simulink model "DALv5"  (R2021b)
settings: Solver=FixedStepAuto  StartTime=0.0  StopTime=100  RelTol=1e-3
undefined symbols (not defined in the file): Beam_Mod, magnitude, N_B, Theta_target, V_wmax
libraries: slpidlib x1
settings Model: ExtModeTrigDuration=2  Creator=Andrea  LastModifiedBy=Andrea
settings OptimizationCC: EnhancedBackFolding=on  PassReuseOutputArgsAs=Individual arguments  ZeroExternalMemoryAtStartup=off  ZeroInternalMemoryAtStartup=off  MaxStackSize=64  OptimizeBlockOrder=speed  DifferentSizesBufferReuse=on  OptimizationCustomize=off  EfficientTunableParamExpr=on
settings DebuggingCC: ParameterTunabilityLossMsg=error
settings HardwareCC: ProdBitPerInt=16  ProdBitPerPointer=16  ProdBitPerSizeT=16  ProdBitPerPtrDiffT=16  ProdLargestAtomicFloat=None  ProdWordSize=8  ProdHWDeviceType=Atmel->AVR
settings SFSimCC: MATLABDynamicMemAlloc=off
settings RTWCC: Description=Embedded Coder  SystemTargetFile=ert.tlc  HardwareBoard=Arduino Uno  TemplateMakefile=ert_default_tmf  Toolchain=Arduino AVR
settings CodeAppCC: ForceParamTrailComments=on  IgnoreCustomStorageClasses=off  OperatorAnnotations=on  SimulinkDataObjDesc=on  SFDataObjDesc=on  InsertBlockDesc=on
settings ERTTargetCC: SupportContinuousTime=on  SupportVariableSizeSignals=on  ExtModeTransport=3  ExtModeStaticAlloc=on  ExtModeStaticAllocSize=250  ExtModeMexFile=ext_xcp  ExtModeIntrfLevel=Level2 - Open

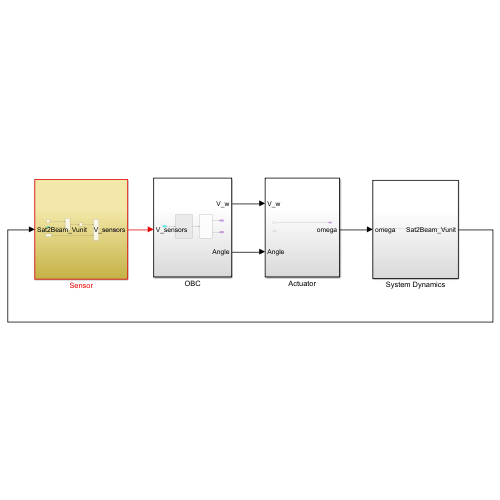
[thumbnail: Simulink's stored preview of the top-level diagram]
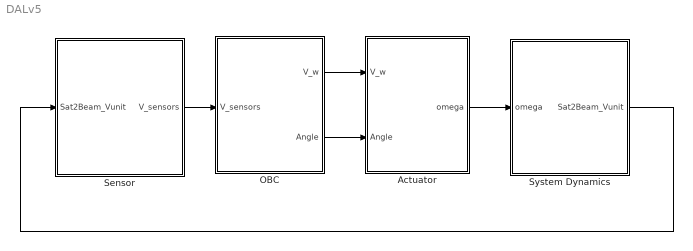
== system DALv5 ==
  Actuator : Subsystem
  OBC : Subsystem
  Sensor : Subsystem
  System Dynamics : Subsystem
  wires:
  System Dynamics/1(Sat2Beam_Vunit) -> Sensor/1(Sat2Beam_Vunit)
  Sensor/1(V_sensors) -> OBC/1(V_sensors)
  OBC/1(V_w) -> Actuator/1(V_w)
  Actuator/1(omega) -> System Dynamics/1(omega)
  OBC/2(Angle) -> Actuator/2(Angle)

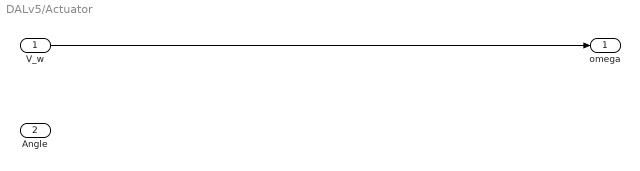
== system DALv5/Actuator ==
  V_w : Inport
  Angle : Inport  Port=2
  omega : Outport
  wires:
  V_w/1 -> omega/1

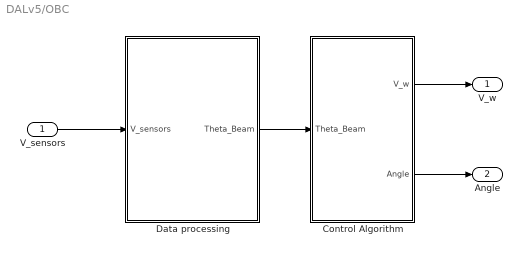
== system DALv5/OBC ==
  V_sensors : Inport
  Control Algorithm : Subsystem
  Data processing : Subsystem
  V_w : Outport
  Angle : Outport  Port=2
  wires:
  V_sensors/1 -> Data processing/1(V_sensors)
  Data processing/1(Theta_Beam) -> Control Algorithm/1(Theta_Beam)
  Control Algorithm/1(V_w) -> V_w/1
  Control Algorithm/2(Angle) -> Angle/1

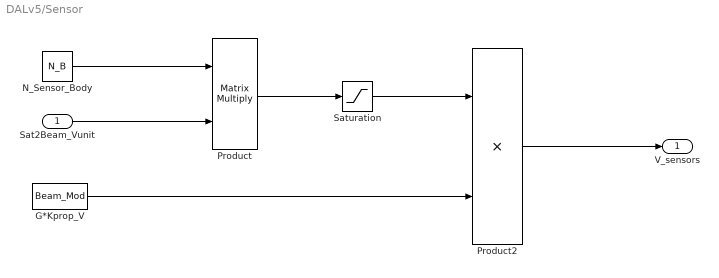
== system DALv5/Sensor ==
  Sat2Beam_Vunit : Inport
  G*Kprop_V : Constant  Value=Beam_Mod
  N_Sensor_Body : Constant  Value=N_B
  Product : Product  Multiplication=Matrix(*)
  Product2 : Product
  Saturation : Saturate  UpperLimit=1  LowerLimit=0
  V_sensors : Outport
  wires:
  Product/1 -> Saturation/1
  N_Sensor_Body/1 -> Product/1
  Saturation/1 -> Product2/1
  Product2/1 -> V_sensors/1
  Sat2Beam_Vunit/1 -> Product/2
  G*Kprop_V/1 -> Product2/2

== system DALv5/System Dynamics ==
  omega : Inport
  Sat2Beam_Vunit : Outport
  wires:
  omega/1 -> Sat2Beam_Vunit/1

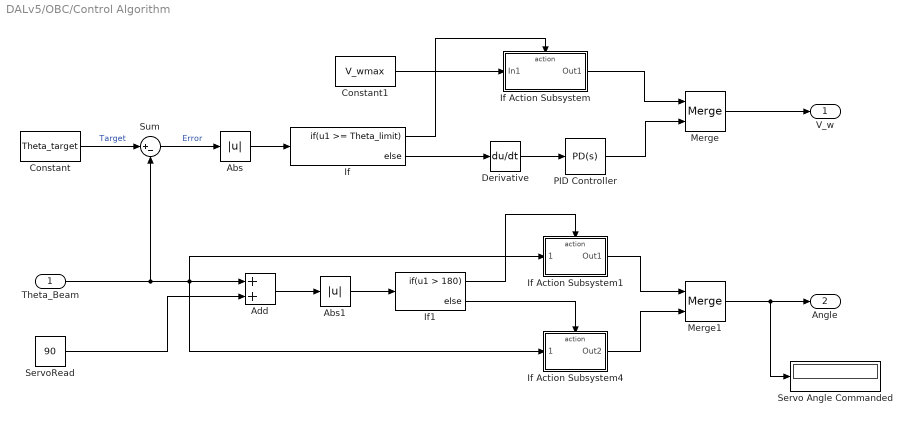
== system DALv5/OBC/Control Algorithm ==
  Theta_Beam : Inport
  Abs : Abs
  Abs1 : Abs
  Add : Sum
  Constant : Constant  Value=Theta_target
  Constant1 : Constant  Value=V_wmax
  Derivative : Derivative
  If : If  IfExpression=u1 >= Theta_limit
  If Action Subsystem : Subsystem  TreatAsAtomicUnit=on
  If Action Subsystem1 : Subsystem  TreatAsAtomicUnit=on
  If Action Subsystem4 : Subsystem  TreatAsAtomicUnit=on
  If1 : If  IfExpression=u1 > 180
  Merge : Merge
  Merge1 : Merge
  PID Controller : slpidlib/PID Controller  Controller=PD  Form=Parallel  TimeDomain=Continuous-time  UseExternalTs=off  SampleTime=-1  IntegratorMethod=Forward Euler  FilterMethod=Forward Euler  ControllerParametersSource=internal  P=1  I=1  D=0  UseFilter=on  N=100  TunerSelectOption=Transfer Function Based (PID Tuner App)  InitialConditionSource=internal  InitialConditionForIntegrator=0  InitialConditionForFilter=0  DifferentiatorICPrevScaledInput=0  ExternalReset=none  TrackingMode=off  Kt=1  LimitOutput=off  SatLimitsSource=internal  UpperSaturationLimit=inf  LowerSaturationLimit=-inf  LinearizeAsGain=on  AntiWindupMode=none  Kb=1  POutMin=[]  POutMax=[]  IOutMin=[]  IOutMax=[]  DOutMin=[]  DOutMax=[]  NOutMin=[]  NOutMax=[]  SumOutMin=[]  SumOutMax=[]  SaturationOutMin=[]  SaturationOutMax=[]  PParamMin=[]  PParamMax=[]  IParamMin=[]  IParamMax=[]  DParamMin=[]  DParamMax=[]  NParamMin=[]  NParamMax=[]  KbParamMin=[]  KbParamMax=[]  KtParamMin=[]  KtParamMax=[]  KbOutMin=[]  KbOutMax=[]  KtOutMin=[]  KtOutMax=[]  IntegratorOutMin=[]  IntegratorOutMax=[]  FilterOutMin=[]  FilterOutMax=[]  SumI1OutMin=[]  SumI1OutMax=[]  SumI2OutMin=[]  SumI2OutMax=[]  SumI3OutMin=[]  SumI3OutMax=[]  SumI4OutMin=[]  SumI4OutMax=[]  SumDOutMin=[]  SumDOutMax=[]  DifferentiatorOutMin=[]  DifferentiatorOutMax=[]  FilterDiffOutCoefMin=[]  FilterDiffOutCoefMax=[]  ReciprocalOutMin=[]  ReciprocalOutMax=[]  SumDenOutMin=[]  SumDenOutMax=[]  SumNumOutMin=[]  SumNumOutMax=[]  DivideOutMin=[]  DivideOutMax=[]  UdiffTsProdOutMin=[]  UdiffTsProdOutMax=[]  NTsProdOutMin=[]  NTsProdOutMax=[]  UintegralTsProdOutMin=[]  UintegralTsProdOutMax=[]  UngainTsProdOutMin=[]  UngainTsProdOutMax=[]  IntegratorContinuousStateAttributes=''  IntegratorStateMustResolveToSignalObject=off  IntegratorRTWStateStorageClass=Auto  FilterContinuousStateAttributes=''  FilterStateMustResolveToSignalObject=off  FilterRTWStateStorageClass=Auto  ParallelPVariant=InternalParameters  IdealPVariant=Disabled  IVariant=Disabled  DVariant=InternalParameters  IntegratorVariant=Disabled  SatVariant=Disabled  AWVariant=Disabled  PCopyVariant=Disabled  TRVariant=Disabled  FdbkBlocksVariant=Forward  IdealPFdbkVariant=Disabled  SatFdbkVariant=Disabled  DerivativeFilterVariant=ContFilter  NVariant=InternalParameters  NCopyVariant=Disabled  FilterICVariant=InternalICsFilter  IntegratorICVariant=Disabled  ExternalResetVariant=Disabled  TRSumVariant=Passthrough  SumFdbkVariant=Disabled  SumVariant=Sum_PD  TsampFilterVariant=InternalTs  TsampNgainVariant=Passthrough  TsampIntegralVariant=Disabled_SignalSpec  ExternalSaturationOutDataTypeStr=Inherit: Same as second input
  Servo Angle Commanded : Display
  ServoRead : Constant  Value=90
  Sum : Sum  Inputs=|+-
  V_w : Outport
  Angle : Outport  Port=2
  wires:
  PID Controller/1 -> Merge/2
  Constant/1 -> Sum/1  "Target"
  Sum/1 -> Abs/1  "Error"
  Constant1/1 -> If Action Subsystem/1(In1)
  If Action Subsystem/1(Out1) -> Merge/1
  If/2 -> Derivative/1
  If/1 -> If Action Subsystem/Action
  Merge/1 -> V_w/1
  Derivative/1 -> PID Controller/1
  Abs/1 -> If/1
  If1/1 -> If Action Subsystem1/Action
  Add/1 -> Abs1/1
  Merge1/1 -> Servo Angle Commanded/1, Angle/1
  Abs1/1 -> If1/1
  Theta_Beam/1 -> If Action Subsystem4/1(Light_Angle), Add/1, If Action Subsystem1/1(Light_Angle), Sum/2
  ServoRead/1 -> Add/2
  If Action Subsystem1/1(Out1) -> Merge1/1
  If1/2 -> If Action Subsystem4/Action
  If Action Subsystem4/1(Out2) -> Merge1/2

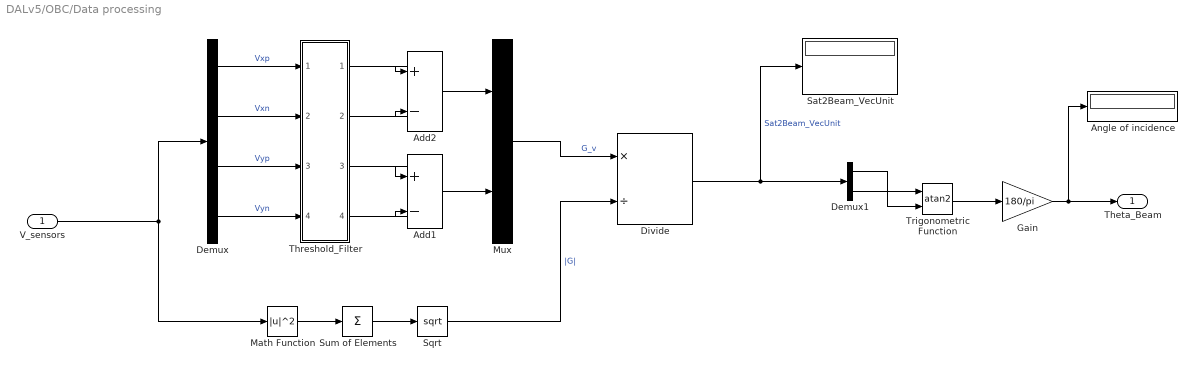
== system DALv5/OBC/Data processing ==
  V_sensors : Inport
  Add1 : Sum  Inputs=+|-
  Add2 : Sum  Inputs=+|-
  Angle of incidence : Display
  Demux : Demux
  Demux1 : Demux  Outputs=2
  Divide : Product  Inputs=*/
  Gain : Gain  Gain=180/pi
  Math Function : Math  Operator=magnitude^2  OutputSignalType=real  SaturateOnIntegerOverflow=on
  Mux : Mux  Inputs=2
  Sat2Beam_VecUnit : Display
  Sqrt : Sqrt  SaturateOnIntegerOverflow=on
  Sum of Elements : Sum  Inputs=+
  Threshold_Filter : Subsystem
  Trigonometric Function : Trigonometry  Operator=atan2
  Theta_Beam : Outport
  wires:
  Threshold_Filter/3(Out3) -> Add1/1
  Threshold_Filter/1(Out1) -> Add2/1
  Threshold_Filter/2(Out2) -> Add2/2
  Demux/4 -> Threshold_Filter/4(Vyn)  "Vyn"
  Demux/2 -> Threshold_Filter/2(Vxn)  "Vxn"
  Demux/1 -> Threshold_Filter/1(Vxp)  "Vxp"
  Demux/3 -> Threshold_Filter/3(Vyp)  "Vyp"
  Threshold_Filter/4(Out4) -> Add1/2
  Math Function/1 -> Sum of Elements/1
  Trigonometric Function/1 -> Gain/1
  Demux1/2 -> Trigonometric Function/1
  Divide/1 -> Demux1/1, Sat2Beam_VecUnit/1  "Sat2Beam_VecUnit"
  Add2/1 -> Mux/1
  Add1/1 -> Mux/2
  Demux1/1 -> Trigonometric Function/2
  Mux/1 -> Divide/1  "G_v"
  V_sensors/1 -> Math Function/1, Demux/1
  Sum of Elements/1 -> Sqrt/1
  Gain/1 -> Angle of incidence/1, Theta_Beam/1
  Sqrt/1 -> Divide/2  "|G|"

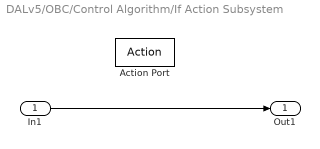
== system DALv5/OBC/Control Algorithm/If Action Subsystem ==
  In1 : Inport
  Action Port : ActionPort  ActionPortLabel=if(u1 <= Theta_limit)
  Out1 : Outport
  wires:
  In1/1 -> Out1/1

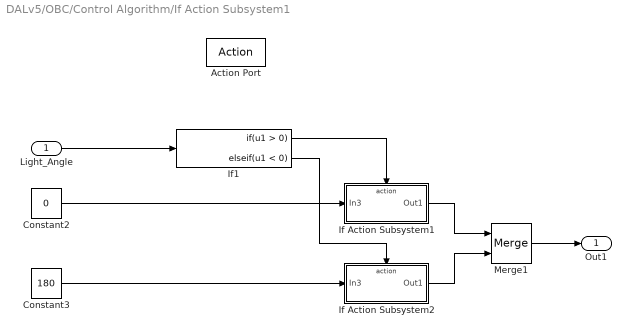
== system DALv5/OBC/Control Algorithm/If Action Subsystem1 ==
  Light_Angle : Inport
  Action Port : ActionPort  ActionPortLabel=if(u1 > 180)
  Constant2 : Constant  Value=0
  Constant3 : Constant  Value=180
  If Action Subsystem1 : Subsystem  TreatAsAtomicUnit=on
  If Action Subsystem2 : Subsystem  TreatAsAtomicUnit=on
  If1 : If  ElseIfExpressions=u1 < 0  ShowElse=off
  Merge1 : Merge
  Out1 : Outport
  wires:
  Light_Angle/1 -> If1/1
  Constant2/1 -> If Action Subsystem1/1(In3)
  Constant3/1 -> If Action Subsystem2/1(In3)
  If1/1 -> If Action Subsystem1/Action
  If1/2 -> If Action Subsystem2/Action
  Merge1/1 -> Out1/1
  If Action Subsystem1/1(Out1) -> Merge1/1
  If Action Subsystem2/1(Out1) -> Merge1/2

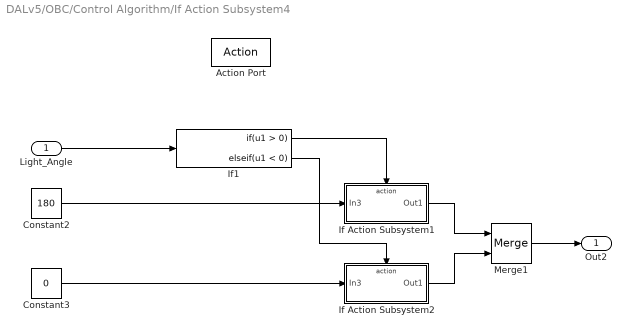
== system DALv5/OBC/Control Algorithm/If Action Subsystem4 ==
  Light_Angle : Inport
  Action Port : ActionPort  ActionPortLabel=else
  Constant2 : Constant  Value=180
  Constant3 : Constant  Value=0
  If Action Subsystem1 : Subsystem  TreatAsAtomicUnit=on
  If Action Subsystem2 : Subsystem  TreatAsAtomicUnit=on
  If1 : If  ElseIfExpressions=u1 < 0  ShowElse=off
  Merge1 : Merge
  Out2 : Outport
  wires:
  If Action Subsystem2/1(Out1) -> Merge1/2
  If1/2 -> If Action Subsystem2/Action
  Merge1/1 -> Out2/1
  Constant2/1 -> If Action Subsystem1/1(In3)
  If Action Subsystem1/1(Out1) -> Merge1/1
  Constant3/1 -> If Action Subsystem2/1(In3)
  If1/1 -> If Action Subsystem1/Action
  Light_Angle/1 -> If1/1

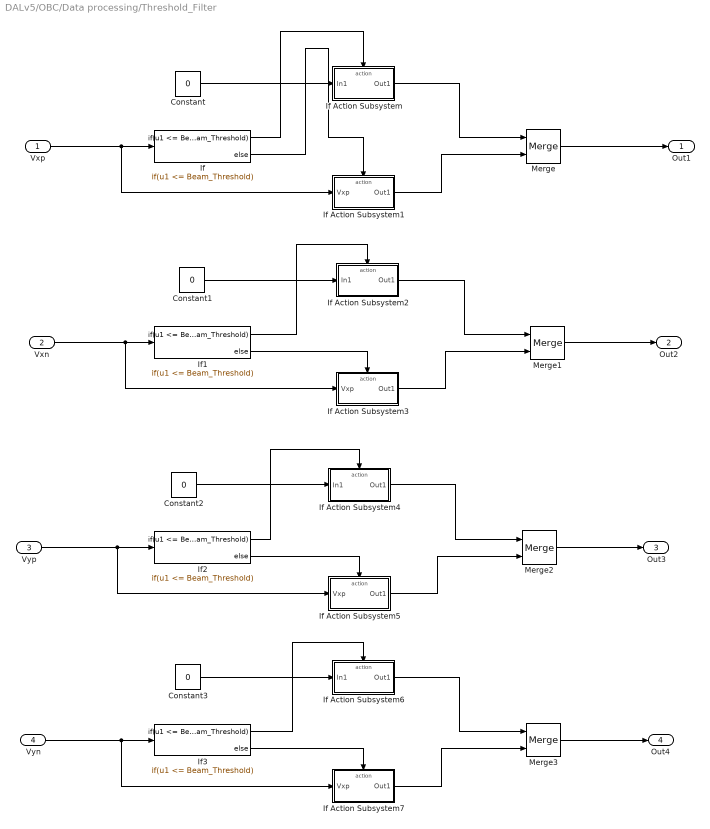
== system DALv5/OBC/Data processing/Threshold_Filter ==
  Vxp : Inport
  Vxn : Inport  Port=2
  Vyp : Inport  Port=3
  Vyn : Inport  Port=4
  Constant{,1..3} (4 alike) : Constant  Value=0
  If{,1..3} (4 alike) : If  IfExpression=u1 <= Beam_Threshold
  If Action Subsystem : Subsystem  TreatAsAtomicUnit=on
  If Action Subsystem1 : Subsystem  TreatAsAtomicUnit=on
  If Action Subsystem2 : Subsystem  TreatAsAtomicUnit=on
  If Action Subsystem3 : Subsystem  TreatAsAtomicUnit=on
  If Action Subsystem4 : Subsystem  TreatAsAtomicUnit=on
  If Action Subsystem5 : Subsystem  TreatAsAtomicUnit=on
  If Action Subsystem6 : Subsystem  TreatAsAtomicUnit=on
  If Action Subsystem7 : Subsystem  TreatAsAtomicUnit=on
  Merge{,1..3} (4 alike) : Merge
  Out1 : Outport
  Out2 : Outport  Port=2
  Out3 : Outport  Port=3
  Out4 : Outport  Port=4
  wires:
  Vxp/1 -> If Action Subsystem1/1(Vxp), If/1
  If/1 -> If Action Subsystem/Action
  If Action Subsystem/1(Out1) -> Merge/1
  If/2 -> If Action Subsystem1/Action
  If Action Subsystem1/1(Out1) -> Merge/2
  Merge/1 -> Out1/1
  Constant/1 -> If Action Subsystem/1(In1)
  If Action Subsystem3/1(Out1) -> Merge1/2
  Constant1/1 -> If Action Subsystem2/1(In1)
  If1/1 -> If Action Subsystem2/Action
  Vxn/1 -> If1/1, If Action Subsystem3/1(Vxp)
  If Action Subsystem2/1(Out1) -> Merge1/1
  If1/2 -> If Action Subsystem3/Action
  Merge1/1 -> Out2/1
  Vyp/1 -> If2/1, If Action Subsystem5/1(Vxp)
  If2/2 -> If Action Subsystem5/Action
  If2/1 -> If Action Subsystem4/Action
  If Action Subsystem4/1(Out1) -> Merge2/1
  If Action Subsystem5/1(Out1) -> Merge2/2
  Constant2/1 -> If Action Subsystem4/1(In1)
  Merge2/1 -> Out3/1
  Vyn/1 -> If3/1, If Action Subsystem7/1(Vxp)
  Merge3/1 -> Out4/1
  If Action Subsystem7/1(Out1) -> Merge3/2
  If3/2 -> If Action Subsystem7/Action
  If Action Subsystem6/1(Out1) -> Merge3/1
  Constant3/1 -> If Action Subsystem6/1(In1)
  If3/1 -> If Action Subsystem6/Action

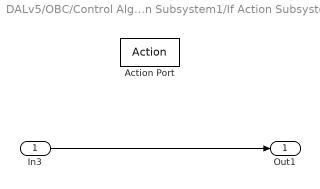
== system DALv5/OBC/Control Algorithm/If Action Subsystem1/If Action Subsystem1 ==
  In3 : Inport
  Action Port : ActionPort
  Out1 : Outport
  wires:
  In3/1 -> Out1/1

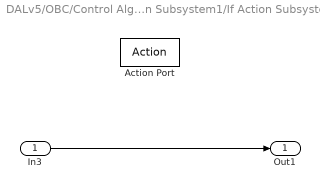
== system DALv5/OBC/Control Algorithm/If Action Subsystem1/If Action Subsystem2 ==
  In3 : Inport
  Action Port : ActionPort
  Out1 : Outport
  wires:
  In3/1 -> Out1/1

== system DALv5/OBC/Control Algorithm/If Action Subsystem4/If Action Subsystem1 ==
  In3 : Inport
  Action Port : ActionPort
  Out1 : Outport
  wires:
  In3/1 -> Out1/1

== system DALv5/OBC/Control Algorithm/If Action Subsystem4/If Action Subsystem2 ==
  In3 : Inport
  Action Port : ActionPort
  Out1 : Outport
  wires:
  In3/1 -> Out1/1

== system DALv5/OBC/Data processing/Threshold_Filter/If Action Subsystem ==
  In1 : Inport
  Action Port : ActionPort  ActionPortLabel=if(u1 <= Beam_Threshold)
  Out1 : Outport
  wires:
  In1/1 -> Out1/1

== system DALv5/OBC/Data processing/Threshold_Filter/If Action Subsystem1 ==
  Vxp : Inport
  Action Port : ActionPort  ActionPortLabel=else
  Out1 : Outport
  wires:
  Vxp/1 -> Out1/1

== system DALv5/OBC/Data processing/Threshold_Filter/If Action Subsystem2 ==
  In1 : Inport
  Action Port : ActionPort  ActionPortLabel=if(u1 <= Beam_Threshold)
  Out1 : Outport
  wires:
  In1/1 -> Out1/1

== system DALv5/OBC/Data processing/Threshold_Filter/If Action Subsystem3 ==
  Vxp : Inport
  Action Port : ActionPort  ActionPortLabel=else
  Out1 : Outport
  wires:
  Vxp/1 -> Out1/1

== system DALv5/OBC/Data processing/Threshold_Filter/If Action Subsystem4 ==
  In1 : Inport
  Action Port : ActionPort  ActionPortLabel=if(u1 <= Beam_Threshold)
  Out1 : Outport
  wires:
  In1/1 -> Out1/1

== system DALv5/OBC/Data processing/Threshold_Filter/If Action Subsystem5 ==
  Vxp : Inport
  Action Port : ActionPort  ActionPortLabel=else
  Out1 : Outport
  wires:
  Vxp/1 -> Out1/1

== system DALv5/OBC/Data processing/Threshold_Filter/If Action Subsystem6 ==
  In1 : Inport
  Action Port : ActionPort  ActionPortLabel=if(u1 <= Beam_Threshold)
  Out1 : Outport
  wires:
  In1/1 -> Out1/1

== system DALv5/OBC/Data processing/Threshold_Filter/If Action Subsystem7 ==
  Vxp : Inport
  Action Port : ActionPort  ActionPortLabel=else
  Out1 : Outport
  wires:
  Vxp/1 -> Out1/1
